simulink model "TestSimpleSfunc"  (R2024b)
settings: Solver=VariableStepAuto  StartTime=0.0  StopTime=10.0  RelTol=1e-3
settings Model: Creator=AdamY  LastModifiedBy=AdamY

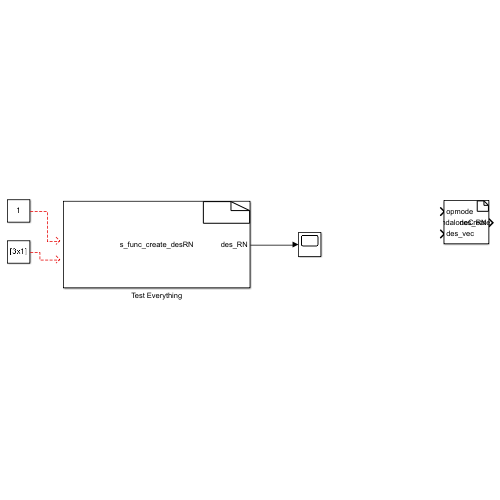
[thumbnail: Simulink's stored preview of the top-level diagram]
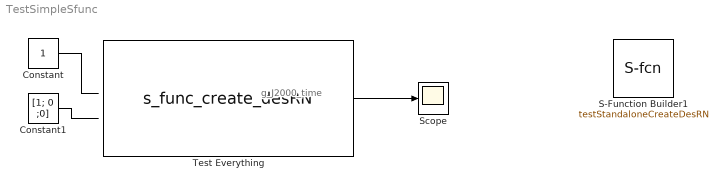
== system TestSimpleSfunc ==
  note: g_J2000_time
  Constant : Constant  OutDataTypeStr=uint8
  Constant1 : Constant  Value=[1; 0 ;0]  OutDataTypeStr=single
  S-Function Builder1 : S-Function  FunctionName=testStandaloneCreateDesRN  SFunctionDeploymentMode=off  EnableBusSupport=off  mask(S-Function Builder){}
      mask help: Simulink:masks:SFunctionBuilder_MD
      mask init:
      | val = [[.9  0.75 0.75 1 1 .9 .9 1]',[1 1 0.75 0.75 .9 .9 1 .9]'];try , sys = get_param(gcb,'SfunBuilderFcnName');if isempty(sys), sys = get_param(gcb,'FunctionName'); end,catch, sys = get_param(gcb,'FunctionName'); end
      settings: CopyFcn=set_param(gcbh,'LinkStatus','none')  OpenFcn=sfunctionwizard(gcbh)
      mask Display: plot(val(:,1),val(:,2)),disp(sys),port_label('input',1,'opmode'),port_label('input',2,'des_vec'),port_label('output',1,'des_RN')
  Scope : Scope
  Test Everything : S-Function  FunctionName=s_func_create_desRN  SFunctionModules=s_func_create_desRN_wrapper.c att_det mtx uart_dbg att conversions ref_rotation global storage pos app uart  SFunctionDeploymentMode=off  EnableBusSupport=off  mask(S-Function Builder){}
      mask help: Simulink:masks:SFunctionBuilder_MD
      mask init: same as TestSimpleSfunc/S-Function Builder1
      settings: CopyFcn=set_param(gcbh,'LinkStatus','none')  OpenFcn=sfunctionwizard(gcbh)
      mask Display: plot(val(:,1),val(:,2)),disp(sys),port_label('output',1,'des_RN')
  wires:
  Constant/1 -> ?
  Constant1/1 -> ?
  Test Everything/1 -> Scope/1
